simulink model "quadcopter_plant"  (R2020b)
settings: Solver=VariableStepAuto  StartTime=0.0  StopTime=10.0  RelTol=1e-3
values from neighbouring files (symbols this model uses):
  dragCoeffMov = 0.01    [iris_quadcopter_specs.m]
  g = 9.81    [iris_quadcopter_specs.m]
  mass = 0.8    [iris_quadcopter_specs.m]
  rotorDir = [-1, -1, 1, 1]    [iris_quadcopter_specs.m]
  rotorPositions = zeros(3,4)    [iris_quadcopter_specs.m]
  rotorThrustMax = 4    [iris_quadcopter_specs.m]
  rotorTimeConst = 0.005    [iris_quadcopter_specs.m]
  rotorTorqueMax = 0.05    [iris_quadcopter_specs.m]
  windVel = [0 0 0]'    [iris_quadcopter_specs.m]
libraries: shared6dof x1
settings Model: Creator=sid  LastModifiedBy=sid

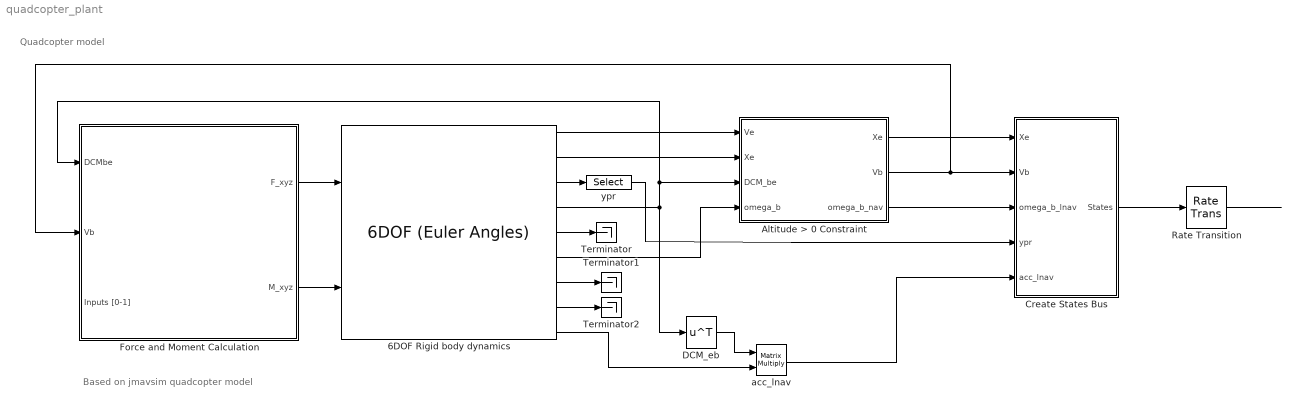
== system quadcopter_plant ==
  note: Quadcopter model
  note: Based on jmavsim quadcopter model
  "6DOF Rigid body dynamics " : shared6dof/6DOF (Euler Angles)  units=Metric (MKS)  mtype=Fixed  rep=Euler Angles  xme_0=init.posNED  Vm_0=init.vb  eul_0=init.euler  pm_0=init.angRates  mass_0=mass  mass_e=0.5  mass_f=2.0  inertia=inertia  inertia_e=eye(3)  inertia_f=2*eye(3)  k_quat=Vehicle.SixDOF.quatGain  vre_flag=on  abi_flag=on  aMode=aMode  xme_statename=''  Vm_statename=''  eul_statename=''  quat_statename=''  pm_statename=''  mass_statename=''
      settings: SourceProductBaseCode=AE,PW,MT,UV,VE,VP
  Altitude > 0 Constraint : MATLAB Function  TreatAsAtomicUnit=on
  Create States Bus : Subsystem
  DCM_eb : Math  Operator=transpose  SaturateOnIntegerOverflow=on
  Force and Moment Calculation : Subsystem
  Rate Transition : RateTransition  OutPortSampleTime=SampleTime
  Terminator : Terminator
  Terminator1 : Terminator
  Terminator2 : Terminator
  acc_lnav : Product  Multiplication=Matrix(*)
  ypr : Selector  InputPortWidth=3  IndexOptions=Index vector (dialog)  Indices=[3 2 1]  OutputSizes=1
  wires:
  "6DOF Rigid body dynamics "/8 -> Terminator2/1
  "6DOF Rigid body dynamics "/7 -> Terminator1/1
  "6DOF Rigid body dynamics "/5 -> Terminator/1
  acc_lnav/1 -> Create States Bus/5(acc_lnav)
  "6DOF Rigid body dynamics "/9 -> acc_lnav/2
  DCM_eb/1 -> acc_lnav/1
  "6DOF Rigid body dynamics "/1 -> Altitude > 0 Constraint/1(Ve)
  "6DOF Rigid body dynamics "/2 -> Altitude > 0 Constraint/2("Xe ")
  Altitude > 0 Constraint/3(omega_b_nav) -> Create States Bus/3(omega_b_lnav)
  "6DOF Rigid body dynamics "/6 -> Altitude > 0 Constraint/4(omega_b)
  Altitude > 0 Constraint/1(Xe) -> Create States Bus/1(Xe)
  "6DOF Rigid body dynamics "/4 -> DCM_eb/1, Force and Moment Calculation/1(DCMbe), Altitude > 0 Constraint/3(DCM_be)
  Create States Bus/1(States) -> Rate Transition/1
  ypr/1 -> Create States Bus/4(ypr)
  ? -> Force and Moment Calculation/3(Inputs [0-1])
  Altitude > 0 Constraint/2(Vb) -> Force and Moment Calculation/2(Vb), Create States Bus/2(Vb)
  Rate Transition/1 -> ?
  Force and Moment Calculation/2(M_xyz) -> "6DOF Rigid body dynamics "/2
  Force and Moment Calculation/1(F_xyz) -> "6DOF Rigid body dynamics "/1
  "6DOF Rigid body dynamics "/3 -> ypr/1

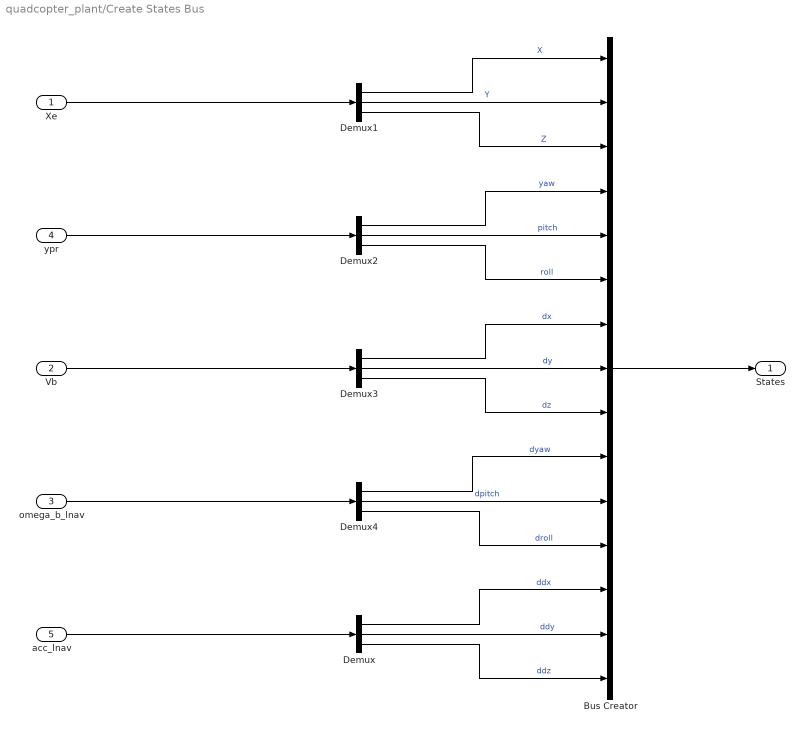
== system quadcopter_plant/Create States Bus ==
  Xe : Inport
  Vb : Inport  Port=2
  omega_b_lnav : Inport  Port=3
  ypr : Inport  Port=4
  acc_lnav : Inport  Port=5
  Bus Creator : BusCreator  Inputs=15
  Demux{,1..4} (5 alike) : Demux  Outputs=3
  States : Outport
  wires:
  Demux1/1 -> Bus Creator/1  "X"
  Demux1/2 -> Bus Creator/2  "Y"
  ypr/1 -> Demux2/1
  Demux2/2 -> Bus Creator/5  "pitch"
  Demux3/2 -> Bus Creator/8  "dy"
  Demux2/3 -> Bus Creator/6  "roll"
  omega_b_lnav/1 -> Demux4/1
  Vb/1 -> Demux3/1
  Demux2/1 -> Bus Creator/4  "yaw"
  Demux1/3 -> Bus Creator/3  "Z"
  Demux3/1 -> Bus Creator/7  "dx"
  Demux4/2 -> Bus Creator/11  "dpitch"
  Demux3/3 -> Bus Creator/9  "dz"
  Demux4/3 -> Bus Creator/12  "droll"
  Demux4/1 -> Bus Creator/10  "dyaw"
  Bus Creator/1 -> States/1
  Xe/1 -> Demux1/1
  acc_lnav/1 -> Demux/1
  Demux/3 -> Bus Creator/15  "ddz"
  Demux/2 -> Bus Creator/14  "ddy"
  Demux/1 -> Bus Creator/13  "ddx"

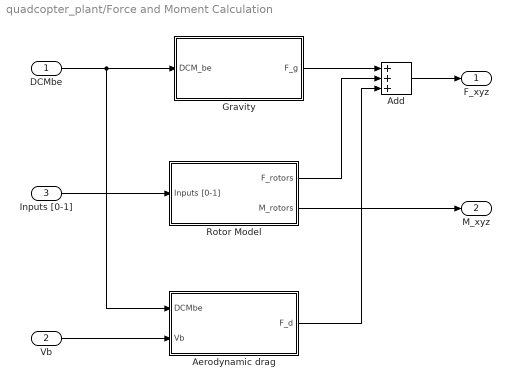
== system quadcopter_plant/Force and Moment Calculation ==
  DCMbe : Inport
  Vb : Inport  Port=2
  Inputs [0-1] : Inport  Port=3
  Add : Sum  Inputs=+++
  Aerodynamic drag : Subsystem
  Gravity : Subsystem
  Rotor Model : Subsystem
  F_xyz : Outport
  M_xyz : Outport  Port=2
  wires:
  Inputs [0-1]/1 -> Rotor Model/1(Inputs [0-1])
  DCMbe/1 -> Aerodynamic drag/1(DCMbe), Gravity/1(DCM_be)
  Gravity/1(F_g) -> Add/1
  Add/1 -> F_xyz/1
  Rotor Model/2(M_rotors) -> M_xyz/1
  Vb/1 -> Aerodynamic drag/2(Vb)
  Rotor Model/1(F_rotors) -> Add/2
  Aerodynamic drag/1(F_d) -> Add/3

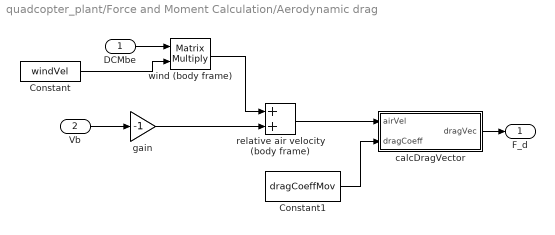
== system quadcopter_plant/Force and Moment Calculation/Aerodynamic drag ==
  DCMbe : Inport
  Vb : Inport  Port=2
  Constant : Constant  Value=windVel
  Constant1 : Constant  Value=dragCoeffMov
  calcDragVector : MATLAB Function  TreatAsAtomicUnit=on
  gain : Gain  Gain=-1
  relative air velocity (body frame) : Sum
  wind (body frame) : Product  Multiplication=Matrix(*)
  F_d : Outport
  wires:
  Vb/1 -> gain/1
  calcDragVector/1(dragVec) -> F_d/1
  relative air velocity (body frame)/1 -> calcDragVector/1(airVel)
  gain/1 -> relative air velocity (body frame)/2
  Constant1/1 -> calcDragVector/2(dragCoeff)
  DCMbe/1 -> wind (body frame)/1
  Constant/1 -> wind (body frame)/2
  wind (body frame)/1 -> relative air velocity (body frame)/1

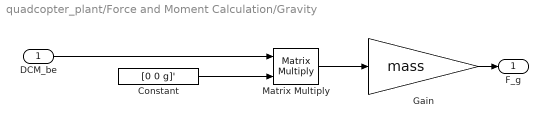
== system quadcopter_plant/Force and Moment Calculation/Gravity ==
  DCM_be : Inport
  Constant : Constant  Value=[0 0 g]'
  Gain : Gain  Gain=mass
  Matrix Multiply : Product  Multiplication=Matrix(*)
  F_g : Outport
  wires:
  Matrix Multiply/1 -> Gain/1
  Constant/1 -> Matrix Multiply/2
  DCM_be/1 -> Matrix Multiply/1
  Gain/1 -> F_g/1

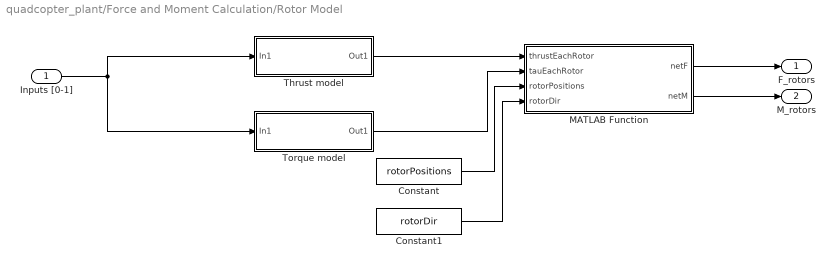
== system quadcopter_plant/Force and Moment Calculation/Rotor Model ==
  Inputs [0-1] : Inport
  Constant : Constant  Value=rotorPositions
  Constant1 : Constant  Value=rotorDir
  MATLAB Function : MATLAB Function  TreatAsAtomicUnit=on
  Thrust model : Subsystem
  Torque model : Subsystem
  F_rotors : Outport
  M_rotors : Outport  Port=2
  wires:
  Inputs [0-1]/1 -> Torque model/1(In1), Thrust model/1(In1)
  MATLAB Function/1(netF) -> F_rotors/1
  MATLAB Function/2(netM) -> M_rotors/1
  Constant/1 -> MATLAB Function/3(rotorPositions)
  Constant1/1 -> MATLAB Function/4(rotorDir)
  Torque model/1(Out1) -> MATLAB Function/2(tauEachRotor)
  Thrust model/1(Out1) -> MATLAB Function/1(thrustEachRotor)

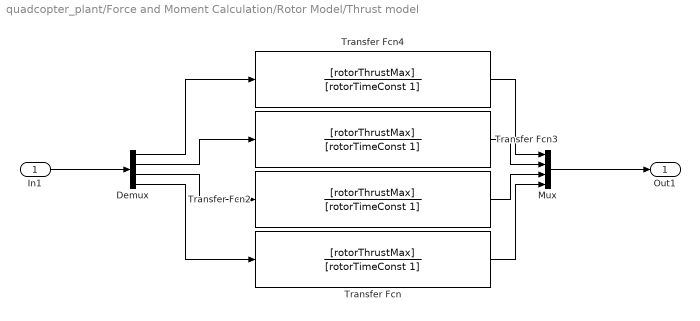
== system quadcopter_plant/Force and Moment Calculation/Rotor Model/Thrust model ==
  In1 : Inport
  Demux : Demux
  Mux : Mux
  Transfer Fcn{,2..4} (4 alike) : TransferFcn  Numerator=[rotorThrustMax]  Denominator=[rotorTimeConst 1]
  Out1 : Outport
  wires:
  Transfer Fcn3/1 -> Mux/2
  Demux/1 -> Transfer Fcn4/1
  Transfer Fcn2/1 -> Mux/3
  Demux/3 -> Transfer Fcn2/1
  Mux/1 -> Out1/1
  Transfer Fcn4/1 -> Mux/1
  Demux/4 -> Transfer Fcn/1
  Demux/2 -> Transfer Fcn3/1
  Transfer Fcn/1 -> Mux/4
  In1/1 -> Demux/1

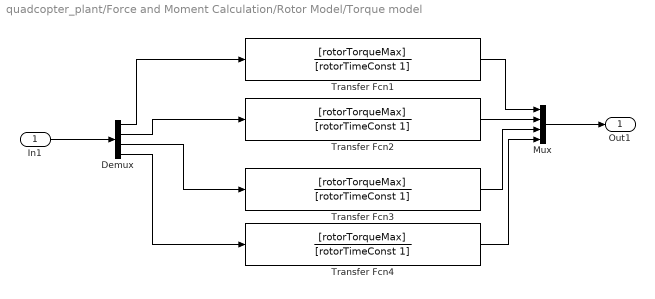
== system quadcopter_plant/Force and Moment Calculation/Rotor Model/Torque model ==
  In1 : Inport
  Demux : Demux
  Mux : Mux
  Transfer Fcn{1..4} (4 alike) : TransferFcn  Numerator=[rotorTorqueMax]  Denominator=[rotorTimeConst 1]
  Out1 : Outport
  wires:
  Transfer Fcn4/1 -> Mux/4
  Demux/1 -> Transfer Fcn1/1
  Transfer Fcn3/1 -> Mux/3
  Transfer Fcn2/1 -> Mux/2
  Demux/2 -> Transfer Fcn2/1
  Demux/4 -> Transfer Fcn4/1
  Demux/3 -> Transfer Fcn3/1
  Mux/1 -> Out1/1
  Transfer Fcn1/1 -> Mux/1
  In1/1 -> Demux/1

== matlab function quadcopter_plant/Force and Moment Calculation/Aerodynamic drag/calcDragVector ==
  data: airVel input; dragVec output; dragCoeff input
function dragVec = fcn(airVel, dragCoeff)

dragVec = dragCoeff * norm(airVel) * airVel;

end

== matlab function quadcopter_plant/Altitude > 0 Constraint ==
  data: Ve input; Xe input; Xe output; Vb output; DCM_be input; omega_b input; omega_b_nav output
function [Xe, Vb, omega_b_nav] = fcn(Ve, Xe, DCM_be, omega_b)
z = Xe(3);
Vz = Ve(3);

if z>=0 && Vz >= 0 %drone on or below gnd and still trying to do down
    Ve = Ve*0; %reset velocity
    omega_b = omega_b*0; %reset omega
    z = 0; % reset height
    Xe(3) = z;
end
% Ve(3) = 0;

Vb = Ve;
omega_b_nav = DCM_be'*omega_b;
end

== matlab function quadcopter_plant/Force and Moment Calculation/Rotor Model/MATLAB Function ==
  data: thrustEachRotor input; tauEachRotor input; rotorPositions input; netF output; netM output; rotorDir input
function [netF, netM] = getForceMoment(thrustEachRotor, tauEachRotor, rotorPositions, rotorDir)
%#codegen
Fx = 0;
Fy = 0;
Fz = -sum(thrustEachRotor);

netF = [Fx; Fy; Fz];

netM = [0; 0; 0]; %initialize
    for i = 1:4
        rotPos = rotorPositions(:, i);
        Fi = [0, 0, -thrustEachRotor(i)]';
        netM = netM +  cross(rotPos, Fi);%contribution from thrusts of each propeller
        netM(3) = netM(3) - rotorDir(i)*tauEachRotor(i); %contribution from counter torque acting on propeller
    end

end
